simulink library "lib_lowLevelController"  (R2023b)
settings: Solver=VariableStepAuto  StartTime=0.0  StopTime=10.0  RelTol=1e-3
settings Model: Creator=muralikarnam  LastModifiedBy=Ruben Rodriguez
settings SolverCC: AlgebraicLoopSolver=TrustRegion
settings DataIOCC: ReturnWorkspaceOutputs=off
settings DebuggingCC: UnconnectedInputMsg=warning  UnconnectedOutputMsg=warning  UnconnectedLineMsg=warning  ArithmeticOperatorsInVariantConditions=warning
settings ModelReferenceCC: EnableRefExpFcnMdlSchedulingChecks=on
settings SFSimCC: SimUseLocalCustomCode=off  CustomCodeUndefinedFunction=UseInterfaceOnly
settings RTWCC: RTWUseLocalCustomCode=off

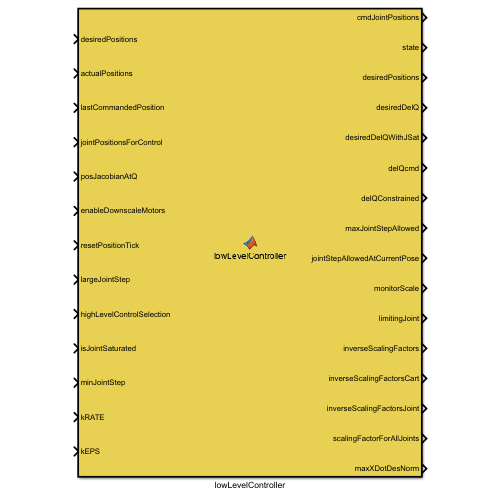
[thumbnail: Simulink's stored preview of the top-level diagram]
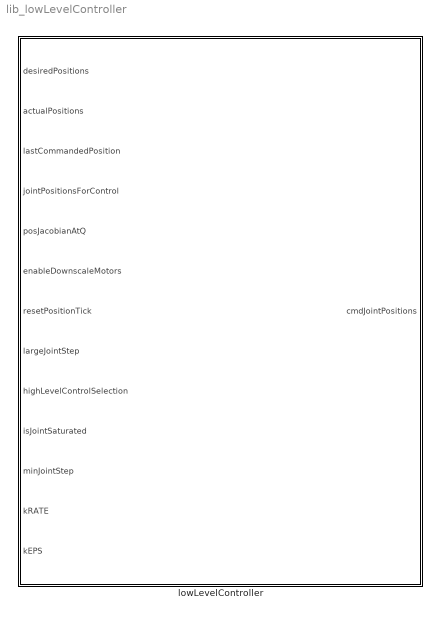
== system lib_lowLevelController ==
  lowLevelController : MATLAB Function  TreatAsAtomicUnit=on

== matlab function lib_lowLevelController/lowLevelController ==
  data: desiredPositions input double size=[nJointsKuka 1]; actualPositions input size=[nJointsKuka 1]; lastCommandedPosition input double size=[nJointsKuka, 1]; jointPositionsForControl input double size=[nJointsKuka 1]; posJacobianAtQ input double size=[3 nJointsKuka nJointsKuka]; enableDownscaleMotors input; resetPositionTick input boolean size=1; largeJointStep input boolean size=1; highLevelControlSelection input uint8 size=1; isJointSaturated input; cmdJointPositions output double size=[nJointsKuka 1]; minJointStep input double size=[2 1]; kRATE input double size=2; kEPS input double size=2; robotParameters parameter Bus: RobotParams
%#codegen
function cmdJointPositions   = lowLevelController(desiredPositions, actualPositions, lastCommandedPosition, jointPositionsForControl, posJacobianAtQ,  enableDownscaleMotors, resetPositionTick, largeJointStep, highLevelControlSelection, isJointSaturated, minJointStep, kRATE, kEPS, robotParameters)


[cmdJointPositions]  = fun_lowLevelController(desiredPositions, actualPositions, lastCommandedPosition, jointPositionsForControl, posJacobianAtQ,  enableDownscaleMotors, resetPositionTick, largeJointStep, highLevelControlSelection, isJointSaturated, minJointStep, kRATE, kEPS, robotParameters);

end
